simulink model "pocetak"  (R2017b)
settings: Solver=VariableStepAuto  StartTime=0.0  StopTime=100  RelTol=1e-3
settings Model: Creator=DT User  LastModifiedBy=DT User

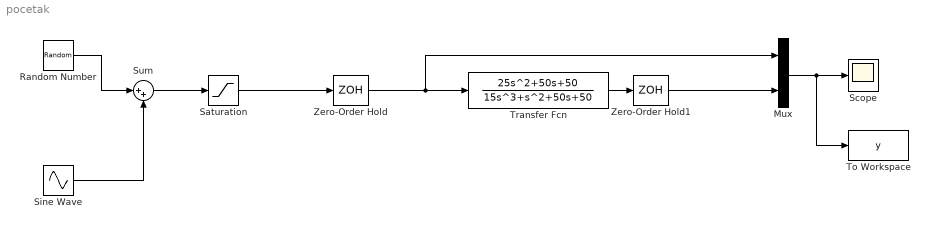
== system pocetak ==
  Mux : Mux  Inputs=2
  Random Number : RandomNumber  Variance=0.1  SampleTime=0.1
  Saturation : Saturate  UpperLimit=5  LowerLimit=-5
  Scope : Scope
  Sine Wave : Sin  Amplitude=4  Frequency=0.0025  SampleTime=0.1
  Sum : Sum  Inputs=|++
  To Workspace : ToWorkspace  VariableName=y  SampleTime=-1
  Transfer Fcn : TransferFcn  Numerator=[25 50 50]  Denominator=[15 1 50 50]
  Zero-Order Hold : ZeroOrderHold  SampleTime=0.1
  Zero-Order Hold1 : ZeroOrderHold  SampleTime=0.1
  wires:
  Sine Wave/1 -> Sum/2
  Random Number/1 -> Sum/1
  Saturation/1 -> Zero-Order Hold/1
  Sum/1 -> Saturation/1
  Zero-Order Hold/1 -> Mux/1, Transfer Fcn/1
  Transfer Fcn/1 -> Zero-Order Hold1/1
  Mux/1 -> To Workspace/1, Scope/1
  Zero-Order Hold1/1 -> Mux/2
